simulink model "model_J"  (R2021b)
settings: Solver=VariableStepAuto  StartTime=0.0  StopTime=1000  RelTol=1e-3
values from neighbouring files (symbols this model uses):
  A = [-6, -25, -35, -10; 0, -9, -15, 0; 0, 6, 9, 0; 4, 17, 26, 6]    [task_1.m]    (also in task_2.m; task_3.m; task_4.m)
  B = [16, 0; 3, 0; -3, 0; -11, 0]    [task_1.m]    (also in task_2.m; task_3.m = [0; 0; 0; 0]; task_4.m)
  C = eye(4)    [task_1.m]    (also in task_2.m; task_3.m = [2, 2, 0, 4; 0, 3, 6, 0]; task_4.m = [2, 2, 0, 4; 0, 3, 6, 0])
  D = zeros(4, 2)    [task_1.m]    (also in task_2.m; task_3.m = zeros(2, 1); task_4.m = [0, 0; 0, 4])
  K_1 = -K_1    [task_1.m]    (also in task_2.m)
  Q_1 = 0.1*eye(4)    [task_1.m]    (also in task_2.m = 0.5*eye(4); task_3.m = inv(eye(4)); task_4.m = eye(4))
  R_1 = 10*eye(2)    [task_1.m]    (also in task_2.m = 0.5*eye(2); task_3.m = inv(10*eye(2)); task_4.m = eye(2))
  x0 = [1000; -1000; 1000; -1000]    [task_1.m]    (also in task_2.m; task_3.m = [10; -10; 5; -5]; task_4.m = [10; -10; 5; -5])
libraries: matrix_library x2
settings Model: Creator=vital  LastModifiedBy=vital

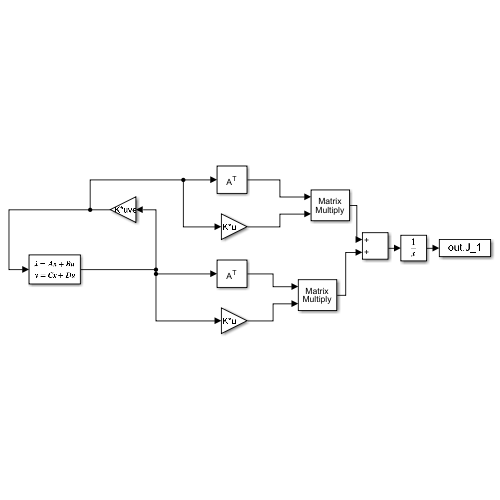
[thumbnail: Simulink's stored preview of the top-level diagram]
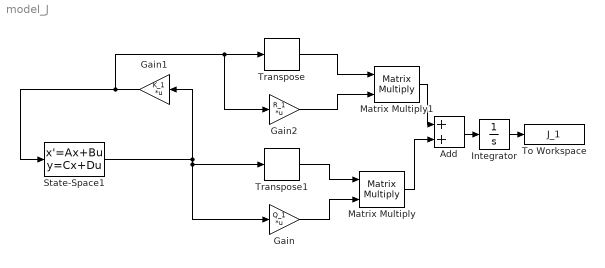
== system model_J ==
  Add : Sum
  Gain : Gain  Gain=Q_1  Multiplication=Matrix(K*u)
  Gain1 : Gain  Gain=K_1  Multiplication=Matrix(K*u) (u vector)
  Gain2 : Gain  Gain=R_1  Multiplication=Matrix(K*u)
  Integrator : Integrator
  Matrix Multiply : Product  Multiplication=Matrix(*)
  Matrix Multiply1 : Product  Multiplication=Matrix(*)
  State-Space1 : StateSpace  A=A  B=B  C=C  D=D  InitialCondition=x0  ParameterTunability=Unconstrained
  To Workspace : ToWorkspace  VariableName=J_1  SaveFormat=Timeseries  SampleTime=0.0001
  Transpose : matrix_library/Transpose
      settings: SourceProductBaseCode=SL
  Transpose1 : matrix_library/Transpose
      settings: SourceProductBaseCode=SL
  wires:
  State-Space1/1 -> Gain/1, Transpose1/1, Gain1/1
  Gain2/1 -> Matrix Multiply1/2
  Transpose/1 -> Matrix Multiply1/1
  Transpose1/1 -> Matrix Multiply/1
  Gain/1 -> Matrix Multiply/2
  Matrix Multiply/1 -> Add/2
  Matrix Multiply1/1 -> Add/1
  Gain1/1 -> Gain2/1, Transpose/1, State-Space1/1
  Add/1 -> Integrator/1
  Integrator/1 -> To Workspace/1
